simulink model "harness"  (Simulink 7.0)
settings: Solver=ode23  StartTime=0.0  StopTime=20  FixedStep=0.01  RelTol=1e-3
InitFcn:
  | init_simulation
StopFcn:
  | post_simulation
values from neighbouring files (symbols this model uses):
  A = pi*R^2    (= 0.0506707479097)    [constants.m]
  accel_noise = noise_on*.01^2    [constants.m]
  Alpha = pi/180*[-85:5:85]    [constants.m]
  att_noise = noise_on*(.25*pi/180)^2    [constants.m]
  att_ref = [0.2 0.2 0 0 0 0]'    [run_simulation.m]
  att_traj_on = 0    [set_scenario.m]
  b = 0.1    [constants.m]
  const_wind = [1 1 0]    [run_simulation.m]
  g = [0 0 9.8]'    [constants.m]
  gyro_noise = noise_on*.01^2    [constants.m]
  J = [Jxx 0 0 ... (first row only)    [constants.m]
  K_a1s = .009    (= 0.009)    [constants.m]
  K_attitude = [  0   kp_p   kp_y     0    kd_p   kd_y ... (first row only)    [run_simulation.m]
  K_beta = 0.23    [constants.m]
  K_dz = 0.7    [run_simulation.m]
  K_flap = 4*(K_beta + T_nom*dz)*K_a1s/(2*dx)    (= 0.0320793572835)    [constants.m]
  K_pz = .37    (= 0.37)    [run_simulation.m]
  K_torque = 0.47    [constants.m]
  M = 1.8263    [constants.m]
  motor_noise = noise_on*(9.8/4*.05)^2    [constants.m]
  plant_int_period = t_s / tau_motor    (= 0.00131578947368)    [constants.m]
  pos_noise = noise_on*0.02^2    [constants.m]
  r1 = [dx 0 -dz]'    [constants.m]
  r2 = [0 dx -dz]'    [constants.m]
  r3 = [-dx 0 -dz]'    [constants.m]
  r4 = [0 -dx -dz]'    [constants.m]
  R_90 = [0 -1 0 ... (first row only)    [constants.m]
  rho = 1.2    [constants.m]
  select = 0    [run_simulation.m]
  T_nom = M*9.8/4    (= 4.474435)    [constants.m]
  t_s = 1/76    (= 0.0131578947368)    [constants.m]
  tau_motor = 10    [constants.m]
  thrust_max = 9.8 * 1    (= 9.8)    [constants.m]
  thrust_min = 0    [constants.m]
  v_min = 1e-3    (= 0.001)    [constants.m]
  vel_noise = noise_on*0.05^2    [constants.m]
  Vh = sqrt(T/(2*rho*A))    [constants.m]
  Vinf = [0:0.5:6]    [constants.m]
  w_seed = 0    [run_simulation.m]
  wind = 3    [run_simulation.m]
  wind_clip = wind_max    (= 10)    [run_simulation.m]
  wind_duration = 5    [run_simulation.m]
  wind_max = 10    [run_simulation.m]
  wind_start = 3    [run_simulation.m]
  wind_var = (wind_max / 10)^2    (= 1)    [run_simulation.m]
  wind_vector = [1 0 0]'    [run_simulation.m]
  zd_ref = 0    [run_simulation.m]
undefined symbols (not defined in the file or in its folder): DiscIntNeverNeededParam, ToverTh
libraries: simulink x20
(part 1 of 3)
settings Model: Creator=Steve  LastModifiedBy=jporter  ExtModeAutoUpdateStatusClock=off
settings DebuggingCC: SaveWithParameterizedLinksMsg=none  SignalResolutionControl=TryResolveAllWithWarning  MultiTaskDSMMsg=warning  MultiTaskCondExecSysMsg=none  StrictBusMsg=None
settings RTWCC: IncludeERTFirstTime=on
settings GRTTargetCC: TargetFcnLib=ansi_tfl_tmw.mat

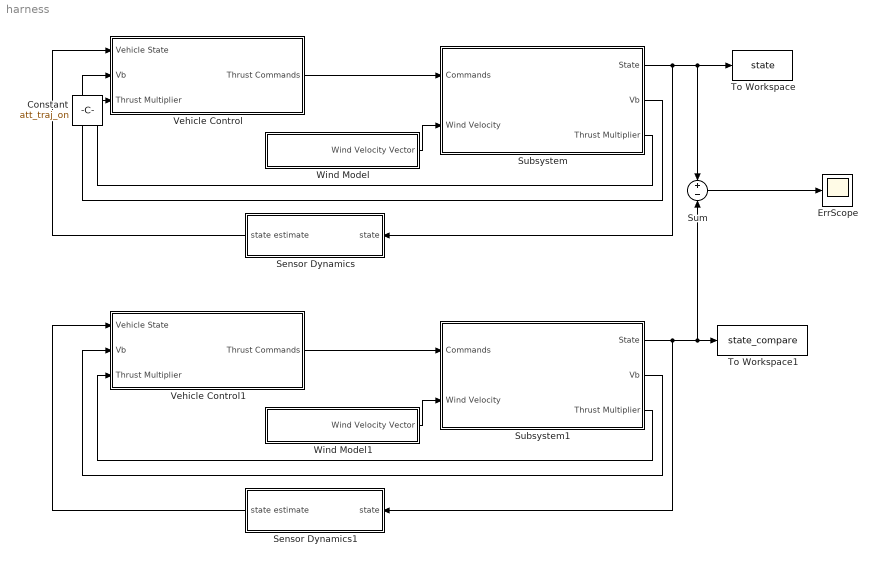
== system harness ==
  ErrScope : Scope
      settings: SaveName=ScopeData22
  Sensor Dynamics : Subsystem  Orientation=left
  Sensor Dynamics1 : Subsystem  Orientation=left
  Subsystem : Subsystem
  Subsystem1 : Subsystem
  Sum : Sum  Inputs=+|-  OutDataType=sfix(16)  OutScaling=2^0
  To Workspace : ToWorkspace  VariableName=state  SampleTime=-1  SaveFormat=Structure With Time
  To Workspace1 : ToWorkspace  VariableName=state_compare  SampleTime=-1  SaveFormat=Structure With Time
  Vehicle Control : Subsystem
  Vehicle Control1 : Subsystem
  Wind Model : Subsystem
  Wind Model1 : Subsystem
  Constant : Constant  IOType=siggen  Value=att_traj_on  OutDataType=sfix(16)  OutScaling=2^0
  wires:
  Wind Model/1(Wind Velocity Vector) -> Subsystem/2(Wind Velocity)
  Vehicle Control/1(Thrust Commands) -> Subsystem/1(Commands)
  Sensor Dynamics/1(state estimate) -> Vehicle Control/1(Vehicle State)
  Subsystem/1(State) -> Sensor Dynamics/1(state), To Workspace/1, Sum/1
  Subsystem/2(Vb) -> Vehicle Control/2(Vb)
  Subsystem/3(Thrust Multiplier) -> Vehicle Control/3(Thrust Multiplier)
  Wind Model1/1(Wind Velocity Vector) -> Subsystem1/2(Wind Velocity)
  Vehicle Control1/1(Thrust Commands) -> Subsystem1/1(Commands)
  Sensor Dynamics1/1(state estimate) -> Vehicle Control1/1(Vehicle State)
  Subsystem1/1(State) -> Sensor Dynamics1/1(state), To Workspace1/1, Sum/2
  Subsystem1/2(Vb) -> Vehicle Control1/2(Vb)
  Subsystem1/3(Thrust Multiplier) -> Vehicle Control1/3(Thrust Multiplier)
  Sum/1 -> ErrScope/1

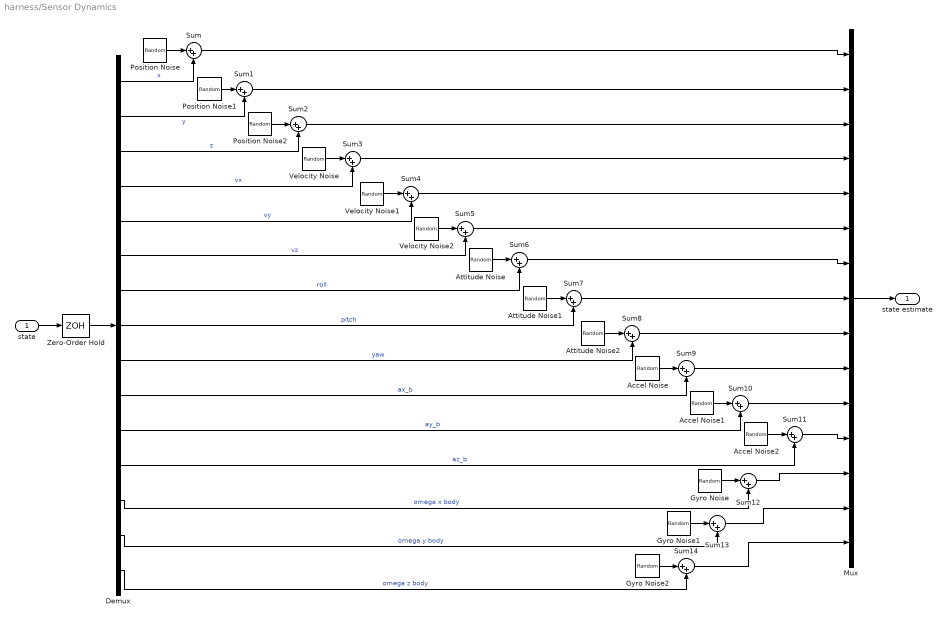
== system harness/Sensor Dynamics ==
  state : Inport  OutDataType=sfix(16)  OutScaling=2^0
  Accel Noise : RandomNumber  Variance=accel_noise  Seed=9  SampleTime=t_s
  Accel Noise1 : RandomNumber  Variance=accel_noise  Seed=10  SampleTime=t_s
  Accel Noise2 : RandomNumber  Variance=accel_noise  Seed=11  SampleTime=t_s
  Attitude Noise : RandomNumber  Variance=att_noise  Seed=6  SampleTime=t_s
  Attitude Noise1 : RandomNumber  Variance=att_noise  Seed=7  SampleTime=t_s
  Attitude Noise2 : RandomNumber  Variance=att_noise  Seed=8  SampleTime=t_s
  Demux : Demux  Outputs=15
  Gyro Noise : RandomNumber  Variance=gyro_noise  Seed=12  SampleTime=t_s
  Gyro Noise1 : RandomNumber  Variance=gyro_noise  Seed=13  SampleTime=t_s
  Gyro Noise2 : RandomNumber  Variance=gyro_noise  Seed=14  SampleTime=t_s
  Mux : Mux  Inputs=15
  Position Noise : RandomNumber  Variance=pos_noise  SampleTime=t_s
  Position Noise1 : RandomNumber  Variance=pos_noise  Seed=1  SampleTime=t_s
  Position Noise2 : RandomNumber  Variance=pos_noise  Seed=3  SampleTime=t_s
  Sum{,1..14} (15 alike) : Sum  Inputs=|++  OutDataType=sfix(16)  OutScaling=2^0
  Velocity Noise : RandomNumber  Variance=vel_noise  Seed=3  SampleTime=t_s
  Velocity Noise1 : RandomNumber  Variance=vel_noise  Seed=4  SampleTime=t_s
  Velocity Noise2 : RandomNumber  Variance=vel_noise  Seed=5  SampleTime=t_s
  Zero-Order Hold : ZeroOrderHold  SampleTime=t_s
  state estimate : Outport  OutDataType=sfix(16)  OutScaling=2^0
  wires:
  state/1 -> Zero-Order Hold/1
  Zero-Order Hold/1 -> Demux/1
  Demux/1 -> Sum/2  "x"
  Demux/2 -> Sum1/2  "y"
  Demux/5 -> Sum4/2  "vy"
  Demux/4 -> Sum3/2  "vx"
  Demux/7 -> Sum6/2  "roll"
  Demux/8 -> Sum7/2  "pitch"
  Demux/9 -> Sum8/2  "yaw"
  Demux/3 -> Sum2/2  "z"
  Demux/6 -> Sum5/2  "vz"
  Demux/10 -> Sum9/2  "ax_b"
  Demux/11 -> Sum10/2  "ay_b"
  Demux/12 -> Sum11/2  "az_b"
  Demux/14 -> Sum13/2  "omega y body"
  Demux/15 -> Sum14/2  "omega z body"
  Demux/13 -> Sum12/2  "omega x body"
  Position Noise/1 -> Sum/1
  Position Noise1/1 -> Sum1/1
  Position Noise2/1 -> Sum2/1
  Velocity Noise/1 -> Sum3/1
  Velocity Noise1/1 -> Sum4/1
  Velocity Noise2/1 -> Sum5/1
  Attitude Noise/1 -> Sum6/1
  Attitude Noise1/1 -> Sum7/1
  Attitude Noise2/1 -> Sum8/1
  Accel Noise/1 -> Sum9/1
  Accel Noise1/1 -> Sum10/1
  Accel Noise2/1 -> Sum11/1
  Gyro Noise/1 -> Sum12/1
  Gyro Noise1/1 -> Sum13/1
  Gyro Noise2/1 -> Sum14/1
  Sum/1 -> Mux/1
  Sum1/1 -> Mux/2
  Sum2/1 -> Mux/3
  Sum3/1 -> Mux/4
  Sum4/1 -> Mux/5
  Sum5/1 -> Mux/6
  Sum6/1 -> Mux/7
  Sum7/1 -> Mux/8
  Sum8/1 -> Mux/9
  Sum9/1 -> Mux/10
  Sum10/1 -> Mux/11
  Sum11/1 -> Mux/12
  Sum12/1 -> Mux/13
  Sum13/1 -> Mux/14
  Sum14/1 -> Mux/15
  Mux/1 -> state estimate/1

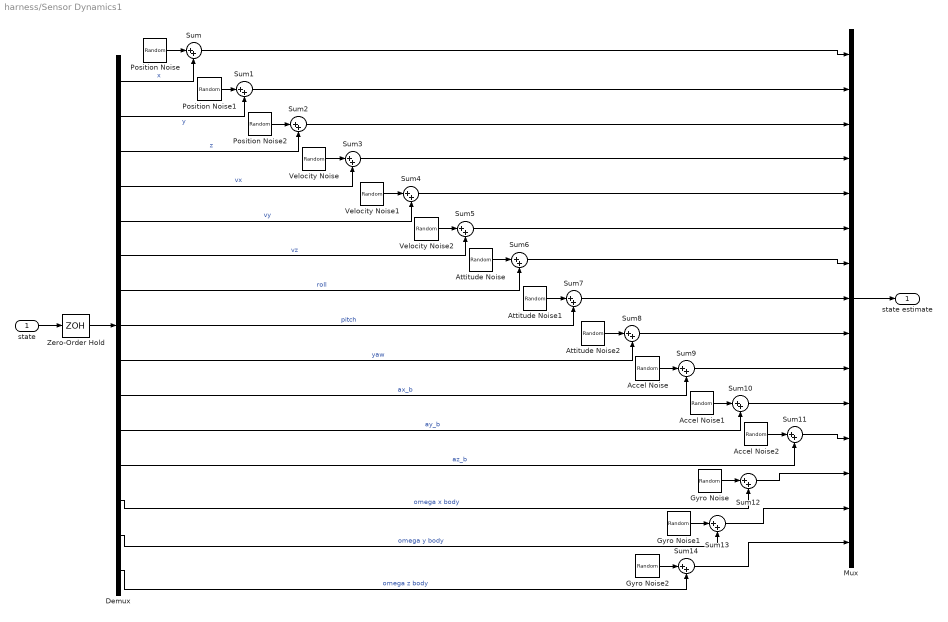
== system harness/Sensor Dynamics1 ==
  state : Inport  OutDataType=sfix(16)  OutScaling=2^0
  Accel Noise : RandomNumber  Variance=accel_noise  Seed=9  SampleTime=t_s
  Accel Noise1 : RandomNumber  Variance=accel_noise  Seed=10  SampleTime=t_s
  Accel Noise2 : RandomNumber  Variance=accel_noise  Seed=11  SampleTime=t_s
  Attitude Noise : RandomNumber  Variance=att_noise  Seed=6  SampleTime=t_s
  Attitude Noise1 : RandomNumber  Variance=att_noise  Seed=7  SampleTime=t_s
  Attitude Noise2 : RandomNumber  Variance=att_noise  Seed=8  SampleTime=t_s
  Demux : Demux  Outputs=15
  Gyro Noise : RandomNumber  Variance=gyro_noise  Seed=12  SampleTime=t_s
  Gyro Noise1 : RandomNumber  Variance=gyro_noise  Seed=13  SampleTime=t_s
  Gyro Noise2 : RandomNumber  Variance=gyro_noise  Seed=14  SampleTime=t_s
  Mux : Mux  Inputs=15
  Position Noise : RandomNumber  Variance=pos_noise  SampleTime=t_s
  Position Noise1 : RandomNumber  Variance=pos_noise  Seed=1  SampleTime=t_s
  Position Noise2 : RandomNumber  Variance=pos_noise  Seed=3  SampleTime=t_s
  Sum{,1..14} (15 alike) : Sum  Inputs=|++  OutDataType=sfix(16)  OutScaling=2^0
  Velocity Noise : RandomNumber  Variance=vel_noise  Seed=3  SampleTime=t_s
  Velocity Noise1 : RandomNumber  Variance=vel_noise  Seed=4  SampleTime=t_s
  Velocity Noise2 : RandomNumber  Variance=vel_noise  Seed=5  SampleTime=t_s
  Zero-Order Hold : ZeroOrderHold  SampleTime=t_s
  state estimate : Outport  OutDataType=sfix(16)  OutScaling=2^0
  wires:
  state/1 -> Zero-Order Hold/1
  Zero-Order Hold/1 -> Demux/1
  Demux/1 -> Sum/2  "x"
  Demux/2 -> Sum1/2  "y"
  Demux/5 -> Sum4/2  "vy"
  Demux/4 -> Sum3/2  "vx"
  Demux/7 -> Sum6/2  "roll"
  Demux/8 -> Sum7/2  "pitch"
  Demux/9 -> Sum8/2  "yaw"
  Demux/3 -> Sum2/2  "z"
  Demux/6 -> Sum5/2  "vz"
  Demux/10 -> Sum9/2  "ax_b"
  Demux/11 -> Sum10/2  "ay_b"
  Demux/12 -> Sum11/2  "az_b"
  Demux/14 -> Sum13/2  "omega y body"
  Demux/15 -> Sum14/2  "omega z body"
  Demux/13 -> Sum12/2  "omega x body"
  Position Noise/1 -> Sum/1
  Position Noise1/1 -> Sum1/1
  Position Noise2/1 -> Sum2/1
  Velocity Noise/1 -> Sum3/1
  Velocity Noise1/1 -> Sum4/1
  Velocity Noise2/1 -> Sum5/1
  Attitude Noise/1 -> Sum6/1
  Attitude Noise1/1 -> Sum7/1
  Attitude Noise2/1 -> Sum8/1
  Accel Noise/1 -> Sum9/1
  Accel Noise1/1 -> Sum10/1
  Accel Noise2/1 -> Sum11/1
  Gyro Noise/1 -> Sum12/1
  Gyro Noise1/1 -> Sum13/1
  Gyro Noise2/1 -> Sum14/1
  Sum/1 -> Mux/1
  Sum1/1 -> Mux/2
  Sum2/1 -> Mux/3
  Sum3/1 -> Mux/4
  Sum4/1 -> Mux/5
  Sum5/1 -> Mux/6
  Sum6/1 -> Mux/7
  Sum7/1 -> Mux/8
  Sum8/1 -> Mux/9
  Sum9/1 -> Mux/10
  Sum10/1 -> Mux/11
  Sum11/1 -> Mux/12
  Sum12/1 -> Mux/13
  Sum13/1 -> Mux/14
  Sum14/1 -> Mux/15
  Mux/1 -> state estimate/1

== system harness/Subsystem ==
  Commands : Inport  OutDataType=sfix(16)  OutScaling=2^0
  Wind Velocity : Inport  Port=2  OutDataType=sfix(16)  OutScaling=2^0
  6DOF (Euler Angles)_CMU : Subsystem
  Aerodynamic Effects : Subsystem
  Gravity : Constant  Value=g * M  OutDataType=sfix(16)  OutScaling=2^0
  Moments : Scope
      settings: SaveName=ScopeData7
  Motor Dynamics : Subsystem
  Mux : Mux  Inputs=5
  Product : Product  Multiplication=Matrix(*)  OutDataType=sfix(16)  OutScaling=2^0  RndMeth=Zero
  Product1 : Product  Multiplication=Matrix(*)  OutDataType=sfix(16)  OutScaling=2^0  RndMeth=Zero
  Sum : Sum  Inputs=|+++  OutDataType=sfix(16)  OutScaling=2^0
  Sum1 : Sum  Inputs=|+-  OutDataType=sfix(16)  OutScaling=2^0
  Terminator : Terminator
  Thrusts actual : Scope
      settings: SaveName=ScopeData9
  Viscous Drag : Gain  Gain=-b  ParameterDataType=sfix(16)  ParameterScaling=2^0  OutDataType=sfix(16)  OutScaling=2^0
  Zero-Order Hold : ZeroOrderHold  SampleTime=t_s
  State : Outport  OutDataType=sfix(16)  OutScaling=2^0
  Vb : Outport  Port=2  OutDataType=sfix(16)  OutScaling=2^0
  Thrust Multiplier : Outport  Port=3  OutDataType=sfix(16)  OutScaling=2^0
  wires:
  Motor Dynamics/1(Motor Thrusts) -> Thrusts actual/1, Aerodynamic Effects/1(Thrusts)
  Product/1 -> Sum/1
  Sum/1 -> 6DOF (Euler Angles)_CMU/1(F_xyz(N))
  6DOF (Euler Angles)_CMU/4(DCM) -> Product/1, Product1/1
  Gravity/1 -> Product/2
  Sum1/1 -> Aerodynamic Effects/2("V (body, relative)"), Viscous Drag/1
  Product1/1 -> Sum1/2
  6DOF (Euler Angles)_CMU/5(Vb) -> Sum1/1, Vb/1
  Viscous Drag/1 -> Sum/3
  6DOF (Euler Angles)_CMU/2(Xe) -> Mux/1
  6DOF (Euler Angles)_CMU/1(Ve) -> Mux/2
  6DOF (Euler Angles)_CMU/3(Euler) -> Mux/3
  Aerodynamic Effects/2(Body Moments) -> Moments/1, 6DOF (Euler Angles)_CMU/2(M_xyz(Nm))
  Aerodynamic Effects/1(Thrust Forces) -> Sum/2
  Zero-Order Hold/1 -> Motor Dynamics/1(Motor Commands)
  Mux/1 -> State/1
  Commands/1 -> Zero-Order Hold/1
  Wind Velocity/1 -> Product1/2
  Aerodynamic Effects/3(Thrust Multiplier) -> Thrust Multiplier/1
  6DOF (Euler Angles)_CMU/7(pdot,qdot,rdot) -> Terminator/1
  6DOF (Euler Angles)_CMU/6(p,q,r) -> Mux/5
  6DOF (Euler Angles)_CMU/8(Ab) -> Mux/4

== system harness/Subsystem1 ==
  Commands : Inport  OutDataType=sfix(16)  OutScaling=2^0
  Wind Velocity : Inport  Port=2  OutDataType=sfix(16)  OutScaling=2^0
  6DOF (Euler Angles)_CMU : Subsystem
  Aerodynamic Effects : Subsystem
  Gravity : Constant  Value=g * M  OutDataType=sfix(16)  OutScaling=2^0
  Moments : Scope
      settings: SaveName=ScopeData7
  Motor Dynamics : Subsystem
  Mux : Mux  Inputs=5
  Product : Product  Multiplication=Matrix(*)  OutDataType=sfix(16)  OutScaling=2^0  RndMeth=Zero
  Product1 : Product  Multiplication=Matrix(*)  OutDataType=sfix(16)  OutScaling=2^0  RndMeth=Zero
  Sum : Sum  Inputs=|+++  OutDataType=sfix(16)  OutScaling=2^0
  Sum1 : Sum  Inputs=|+-  OutDataType=sfix(16)  OutScaling=2^0
  Terminator : Terminator
  Thrusts actual : Scope
      settings: SaveName=ScopeData9
  Viscous Drag : Gain  Gain=-b  ParameterDataType=sfix(16)  ParameterScaling=2^0  OutDataType=sfix(16)  OutScaling=2^0
  Zero-Order Hold : ZeroOrderHold  SampleTime=plant_int_period
  State : Outport  OutDataType=sfix(16)  OutScaling=2^0
  Vb : Outport  Port=2  OutDataType=sfix(16)  OutScaling=2^0
  Thrust Multiplier : Outport  Port=3  OutDataType=sfix(16)  OutScaling=2^0
  wires:
  Motor Dynamics/1(Motor Thrusts) -> Thrusts actual/1, Aerodynamic Effects/1(Thrusts)
  Product/1 -> Sum/1
  Sum/1 -> 6DOF (Euler Angles)_CMU/1(F_xyz(N))
  6DOF (Euler Angles)_CMU/4(DCM) -> Product/1, Product1/1
  Gravity/1 -> Product/2
  Sum1/1 -> Aerodynamic Effects/2("V (body, relative)"), Viscous Drag/1
  Product1/1 -> Sum1/2
  6DOF (Euler Angles)_CMU/5(Vb) -> Sum1/1, Vb/1
  Viscous Drag/1 -> Sum/3
  6DOF (Euler Angles)_CMU/2(Xe) -> Mux/1
  6DOF (Euler Angles)_CMU/1(Ve) -> Mux/2
  6DOF (Euler Angles)_CMU/3(Euler) -> Mux/3
  Aerodynamic Effects/2(Body Moments) -> Moments/1, 6DOF (Euler Angles)_CMU/2(M_xyz(Nm))
  Aerodynamic Effects/1(Thrust Forces) -> Sum/2
  Mux/1 -> State/1
  Commands/1 -> Motor Dynamics/1(Motor Commands)
  Wind Velocity/1 -> Zero-Order Hold/1
  Aerodynamic Effects/3(Thrust Multiplier) -> Thrust Multiplier/1
  6DOF (Euler Angles)_CMU/7(pdot,qdot,rdot) -> Terminator/1
  6DOF (Euler Angles)_CMU/6(p,q,r) -> Mux/5
  6DOF (Euler Angles)_CMU/8(Ab) -> Mux/4
  Zero-Order Hold/1 -> Product1/2

== system harness/Vehicle Control ==
  Vehicle State : Inport  OutDataType=sfix(16)  OutScaling=2^0
  Vb : Inport  Port=2  OutDataType=sfix(16)  OutScaling=2^0
  Thrust Multiplier : Inport  Port=3  OutDataType=sfix(16)  OutScaling=2^0
  Altitude Control : Subsystem
  Attitude Control : Subsystem
  Position Control : Subsystem
  Reference Altitude : FromWorkspace  VariableName=alt_traj  SampleTime=0
  Reference Attitude : FromWorkspace  VariableName=att_traj  SampleTime=0
  Scope : Scope
      settings: SaveName=ScopeData11
  Scope1 : Scope
      settings: SaveName=ScopeData12
  Sum : Sum  Inputs=|++  OutDataType=sfix(16)  OutScaling=2^0
  Switch : Switch
  Thrust Commands : Outport  OutDataType=sfix(16)  OutScaling=2^0
  wires:
  Vehicle State/1 -> Position Control/1(state), Attitude Control/2(State), Altitude Control/2(state)
  Attitude Control/1(Thrusts) -> Sum/1
  Position Control/1(Attitude) -> Switch/3
  Switch/1 -> Attitude Control/1(Attitude Commands)
  Reference Attitude/1 -> Scope/1, Switch/1
  Sum/1 -> Thrust Commands/1
  Altitude Control/1(commands) -> Sum/2
  Reference Altitude/1 -> Scope1/1, Altitude Control/1(altitude  commands)
  Vb/1 -> Attitude Control/3(Vb)
  Thrust Multiplier/1 -> Altitude Control/3(Thrust Multiplier)

== system harness/Vehicle Control1 ==
  Vehicle State : Inport  OutDataType=sfix(16)  OutScaling=2^0
  Vb : Inport  Port=2  OutDataType=sfix(16)  OutScaling=2^0
  Thrust Multiplier : Inport  Port=3  OutDataType=sfix(16)  OutScaling=2^0
  Altitude Control : Subsystem
  Attitude Control : Subsystem
  Constant : Constant  Value=att_traj_on  OutDataType=sfix(16)  OutScaling=2^0
  Position Control : Subsystem
  Reference Altitude : FromWorkspace  VariableName=alt_traj  SampleTime=0
  Reference Attitude : FromWorkspace  VariableName=att_traj  SampleTime=0
  Scope : Scope
      settings: SaveName=ScopeData11
  Scope1 : Scope
      settings: SaveName=ScopeData12
  Sum : Sum  Inputs=|++  OutDataType=sfix(16)  OutScaling=2^0
  Switch : Switch
  Zero-Order Hold : ZeroOrderHold  SampleTime=t_s
  Thrust Commands : Outport  OutDataType=sfix(16)  OutScaling=2^0
  wires:
  Vehicle State/1 -> Position Control/1(state), Attitude Control/2(State), Altitude Control/2(state)
  Attitude Control/1(Thrusts) -> Sum/1
  Position Control/1(Attitude) -> Switch/3
  Switch/1 -> Attitude Control/1(Attitude Commands)
  Reference Attitude/1 -> Switch/1, Scope/1
  Sum/1 -> Zero-Order Hold/1
  Altitude Control/1(commands) -> Sum/2
  Reference Altitude/1 -> Scope1/1, Altitude Control/1(altitude  commands)
  Vb/1 -> Attitude Control/3(Vb)
  Thrust Multiplier/1 -> Altitude Control/3(Thrust Multiplier)
  Zero-Order Hold/1 -> Thrust Commands/1
  Constant/1 -> Switch/2

== system harness/Wind Model ==
  Constant : Constant  Value=wind  OutDataType=sfix(16)  OutScaling=2^0
  Constant wind : Constant  Value=const_wind  OutDataType=sfix(16)  OutScaling=2^0
  Multiport Switch : MultiPortSwitch  Inputs=3
  Single Wind Gust Model : Subsystem  TreatAsAtomicUnit=on
  Step : Step  Time=wind_start  SampleTime=0
  Step1 : Step  Time=wind_start+wind_duration  After=-1  SampleTime=0
  Sum : Sum  Inputs=|++  OutDataType=sfix(16)  OutScaling=2^0
  Zero Wind : Constant  Value=[0 0 0]'  OutDataType=sfix(16)  OutScaling=2^0
  wind : Scope
      settings: SaveName=ScopeData4
  Wind Velocity Vector : Outport  OutDataType=sfix(16)  OutScaling=2^0
  wires:
  Multiport Switch/1 -> Wind Velocity Vector/1, wind/1
  Step/1 -> Sum/1  "start"
  Step1/1 -> Sum/2  "stop"
  Sum/1 -> Single Wind Gust Model/Enable
  Constant/1 -> Multiport Switch/1
  Zero Wind/1 -> Multiport Switch/2
  Constant wind/1 -> Multiport Switch/3
  Single Wind Gust Model/1(Wind Velocity) -> Multiport Switch/4

== system harness/Wind Model1 ==
  Constant : Constant  Value=wind  OutDataType=sfix(16)  OutScaling=2^0
  Constant wind : Constant  Value=const_wind  OutDataType=sfix(16)  OutScaling=2^0
  Multiport Switch : MultiPortSwitch  Inputs=3
  Single Wind Gust Model : Subsystem  TreatAsAtomicUnit=on
  Step : Step  Time=wind_start  SampleTime=0
  Step1 : Step  Time=wind_start+wind_duration  After=-1  SampleTime=0
  Sum : Sum  Inputs=|++  OutDataType=sfix(16)  OutScaling=2^0
  Zero Wind : Constant  Value=[0 0 0]'  OutDataType=sfix(16)  OutScaling=2^0
  wind : Scope
      settings: SaveName=ScopeData4
  Wind Velocity Vector : Outport  OutDataType=sfix(16)  OutScaling=2^0
  wires:
  Multiport Switch/1 -> Wind Velocity Vector/1, wind/1
  Step/1 -> Sum/1  "start"
  Step1/1 -> Sum/2  "stop"
  Sum/1 -> Single Wind Gust Model/Enable
  Constant/1 -> Multiport Switch/1
  Zero Wind/1 -> Multiport Switch/2
  Constant wind/1 -> Multiport Switch/3
  Single Wind Gust Model/1(Wind Velocity) -> Multiport Switch/4

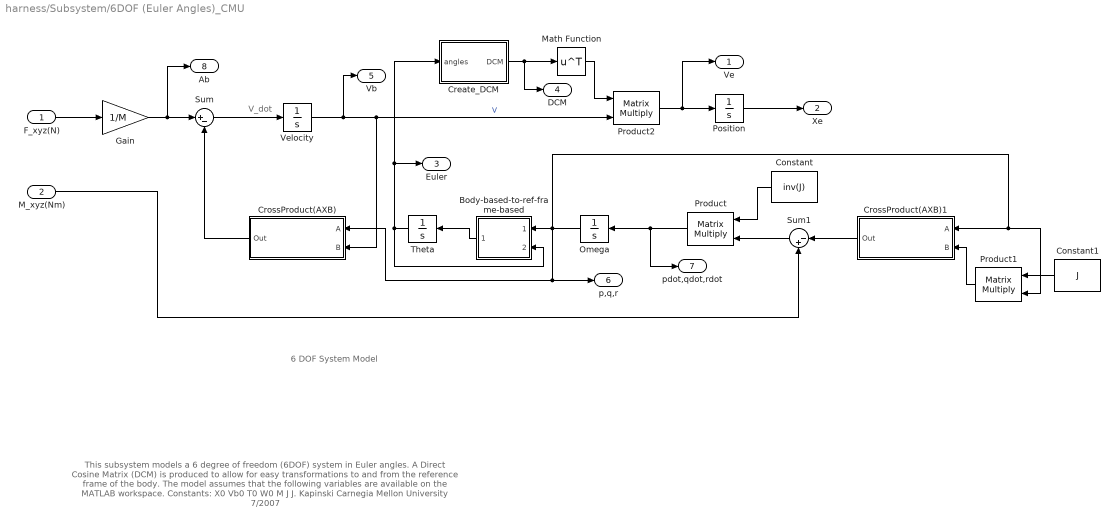
== system harness/Subsystem/6DOF (Euler Angles)_CMU ==
  note: 6 DOF System Model
  note: V_dot
  note: This subsystem models a 6 degree of freedom (6DOF) system in Euler angles.
      | A Direct Cosine Matrix (DCM) is produced to allow for easy transformations to
      | and from the reference frame of the body.  The model assumes that the
      | following variables are available on the MATLAB workspace.
      |
      | Constants:
      | X0
      | Vb0
      | T0
      | W0
      | M
      | J
      |
      | J. Kapinski
      | Carnegia Mellon University
      | 7/2007
  F_xyz(N) : Inport  OutDataType=sfix(16)  OutScaling=2^0
  M_xyz(Nm) : Inport  Port=2  PortDimensions=3  OutDataType=sfix(16)  OutScaling=2^0
  Body-based-to-ref-frame-based : Subsystem  Orientation=left
  Constant : Constant  Orientation=left  Value=inv(J)  OutDataType=sfix(16)  OutScaling=2^0
  Constant1 : Constant  Orientation=left  Value=J  OutDataType=sfix(16)  OutScaling=2^0
  Create_DCM : Subsystem
  CrossProduct(AXB) : Subsystem  Orientation=left
  CrossProduct(AXB)1 : Subsystem  Orientation=left
  Gain : Gain  Gain=1/M  ParameterDataType=sfix(16)  ParameterScaling=2^0  OutDataType=sfix(16)  OutScaling=2^0
  Math Function : Math  Operator=transpose  OutDataType=sfix(16)  OutScaling=2^0  SaturateOnIntegerOverflow=on
  Omega : Integrator  Orientation=left
  Position : Integrator
  Product : Product  Orientation=left  Multiplication=Matrix(*)  OutDataType=sfix(16)  OutScaling=2^0  RndMeth=Zero
  Product1 : Product  Orientation=left  Multiplication=Matrix(*)  OutDataType=sfix(16)  OutScaling=2^0  RndMeth=Zero
  Product2 : Product  Multiplication=Matrix(*)  OutDataType=sfix(16)  OutScaling=2^0  RndMeth=Zero
  Sum : Sum  Inputs=|+-  OutDataType=sfix(16)  OutScaling=2^0
  Sum1 : Sum  Orientation=left  Inputs=|-+  OutDataType=sfix(16)  OutScaling=2^0
  Theta : Integrator  Orientation=left
  Velocity : Integrator
  Ve : Outport  OutDataType=sfix(16)  OutScaling=2^0
  Xe : Outport  Port=2  OutDataType=sfix(16)  OutScaling=2^0
  Euler : Outport  Port=3  OutDataType=sfix(16)  OutScaling=2^0
  DCM : Outport  Port=4  OutDataType=sfix(16)  OutScaling=2^0
  Vb : Outport  Port=5  OutDataType=sfix(16)  OutScaling=2^0
  p,q,r : Outport  Port=6  OutDataType=sfix(16)  OutScaling=2^0
  pdot,qdot,rdot : Outport  Port=7  OutDataType=sfix(16)  OutScaling=2^0
  Ab : Outport  Port=8  OutDataType=sfix(16)  OutScaling=2^0
  wires:
  Position/1 -> Xe/1
  Product2/1 -> Ve/1, Position/1
  Math Function/1 -> Product2/1
  Create_DCM/1(DCM) -> DCM/1, Math Function/1
  Body-based-to-ref-frame-based/1(Out1) -> Theta/1
  Theta/1 -> Euler/1, Create_DCM/1(angles), Body-based-to-ref-frame-based/2(theta)
  Product1/1 -> CrossProduct(AXB)1/2(B)
  Constant1/1 -> Product1/1
  CrossProduct(AXB)1/1(Out) -> Sum1/1
  M_xyz(Nm)/1 -> Sum1/2
  Sum1/1 -> Product/2
  Product/1 -> pdot,qdot,rdot/1, Omega/1
  Constant/1 -> Product/1
  Velocity/1 -> Vb/1, Product2/2, CrossProduct(AXB)/2(B)  "V"
  Omega/1 -> p,q,r/1, CrossProduct(AXB)/1(A), Body-based-to-ref-frame-based/1(omega), Product1/2, CrossProduct(AXB)1/1(A)
  Sum/1 -> Velocity/1
  CrossProduct(AXB)/1(Out) -> Sum/2
  Gain/1 -> Ab/1, Sum/1
  F_xyz(N)/1 -> Gain/1

== system harness/Subsystem/Aerodynamic Effects ==
  Thrusts : Inport  OutDataType=sfix(16)  OutScaling=2^0
  "V (body, relative)" : Inport  Port=2  OutDataType=sfix(16)  OutScaling=2^0
  Flapping Dynamics : Subsystem
  Moments : Subsystem
  Pick First 2 Elements : Constant  Value=[1 0 0; 0 1 0; 0 0 0]  OutDataType=sfix(16)  OutScaling=2^0
  Product : Product  OutDataType=sfix(16)  OutScaling=2^0  RndMeth=Zero
  Product2 : Product  Multiplication=Matrix(*)  OutDataType=sfix(16)  OutScaling=2^0  RndMeth=Zero
  Product4 : Product  OutDataType=sfix(16)  OutScaling=2^0  RndMeth=Zero
  Sum : Sum  Inputs=|++  OutDataType=sfix(16)  OutScaling=2^0
  Sum of Elements : Sum  Inputs=+  OutDataType=sfix(16)  OutScaling=2^-10
  Vertical Effect Dynamics : Subsystem
  Thrust Forces : Outport  OutDataType=sfix(16)  OutScaling=2^0
  Body Moments : Outport  Port=2  OutDataType=sfix(16)  OutScaling=2^0
  Thrust Multiplier : Outport  Port=3  OutDataType=sfix(16)  OutScaling=2^0
  wires:
  Thrusts/1 -> Product/1, Vertical Effect Dynamics/1(Thrust Command)
  Vertical Effect Dynamics/1(Thrust Multiplier) -> Product/2, Thrust Multiplier/1
  Product/1 -> Sum of Elements/1, Moments/1(Thrust Magnitudes)
  Pick First 2 Elements/1 -> Product2/1
  "V (body, relative)"/1 -> Product2/2, Vertical Effect Dynamics/2(V (body))
  Product2/1 -> Flapping Dynamics/1(Vb2_hat)
  Sum of Elements/1 -> Product4/1
  Product4/1 -> Thrust Forces/1
  Flapping Dynamics/1(thrust vector) -> Moments/2(Thrust Vector), Product4/2
  Moments/1(Body Moments) -> Sum/1
  Sum/1 -> Body Moments/1
  Flapping Dynamics/2(rotor blade moments) -> Sum/2

== system harness/Subsystem/Motor Dynamics ==
  Motor Commands : Inport  OutDataType=sfix(16)  OutScaling=2^0
  Demux : Demux
  Motor Noise Source : Subsystem
  Mux : Mux
  Saturation{,1..3} (4 alike) : Saturate  UpperLimit=thrust_max  LowerLimit=thrust_min
  Scope : Scope
      settings: SaveName=ScopeData8
  State-Space : StateSpace  A=-tau_motor*eye(4)  B=tau_motor*eye(4)  C=eye(4)  D=zeros(4,4)  X0=T_nom*ones(4,1)
  Sum{,1..3} (4 alike) : Sum  Inputs=|++  OutDataType=sfix(16)  OutScaling=2^0
  Motor Thrusts : Outport  OutDataType=sfix(16)  OutScaling=2^0
  wires:
  Demux/1 -> Saturation/1
  Demux/3 -> Saturation2/1
  Mux/1 -> Motor Thrusts/1
  Saturation/1 -> Sum/1
  Sum/1 -> Mux/1
  Saturation1/1 -> Sum2/1
  Sum2/1 -> Mux/2
  Saturation2/1 -> Sum3/1
  Sum3/1 -> Mux/3
  Saturation3/1 -> Sum1/1
  Sum1/1 -> Mux/4
  Motor Noise Source/1(Motor 1) -> Sum/2
  Motor Noise Source/2(Motor 2) -> Sum2/2
  Motor Noise Source/3(Motor 3) -> Sum3/2
  Motor Noise Source/4(Motor 4) -> Sum1/2
  Motor Commands/1 -> State-Space/1, Scope/1
  State-Space/1 -> Demux/1
  Demux/2 -> Saturation1/1
  Demux/4 -> Saturation3/1

== system harness/Subsystem1/6DOF (Euler Angles)_CMU ==
  note: 6 DOF System Model
  note: V_dot
  note: This subsystem models a 6 degree of freedom (6DOF) system in Euler angles.
      | A Direct Cosine Matrix (DCM) is produced to allow for easy transformations to
      | and from the reference frame of the body.  The model assumes that the
      | following variables are available on the MATLAB workspace.
      |
      | Constants:
      | X0
      | Vb0
      | T0
      | W0
      | M
      | J
      |
      | J. Kapinski
      | Carnegia Mellon University
      | 7/2007
  F_xyz(N) : Inport  OutDataType=sfix(16)  OutScaling=2^0
  M_xyz(Nm) : Inport  Port=2  PortDimensions=3  OutDataType=sfix(16)  OutScaling=2^0
  Body-based-to-ref-frame-based : Subsystem  Orientation=left
  Constant : Constant  Orientation=left  Value=inv(J)  OutDataType=sfix(16)  OutScaling=2^0
  Constant1 : Constant  Orientation=left  Value=J  OutDataType=sfix(16)  OutScaling=2^0
  Create_DCM : Subsystem
  CrossProduct(AXB) : Subsystem  Orientation=left
  CrossProduct(AXB)1 : Subsystem  Orientation=left
  Discrete-Time Omega : DiscreteIntegrator  Orientation=left  SampleTime=plant_int_period  OutDataType=sfix(16)  OutScaling=2^0  ICPrevOutput=DiscIntNeverNeededParam  ICPrevScaledInput=DiscIntNeverNeededParam
  Discrete-Time Position : DiscreteIntegrator  SampleTime=plant_int_period  OutDataType=sfix(16)  OutScaling=2^0  ICPrevOutput=DiscIntNeverNeededParam  ICPrevScaledInput=DiscIntNeverNeededParam
  Discrete-Time Theta : DiscreteIntegrator  Orientation=left  SampleTime=plant_int_period  OutDataType=sfix(16)  OutScaling=2^0  ICPrevOutput=DiscIntNeverNeededParam  ICPrevScaledInput=DiscIntNeverNeededParam
  Discrete-Time Velocity : DiscreteIntegrator  SampleTime=plant_int_period  OutDataType=sfix(16)  OutScaling=2^0  ICPrevOutput=DiscIntNeverNeededParam  ICPrevScaledInput=DiscIntNeverNeededParam
  Gain : Gain  Gain=1/M  ParameterDataType=sfix(16)  ParameterScaling=2^0  OutDataType=sfix(16)  OutScaling=2^0
  Math Function : Math  Operator=transpose  OutDataType=sfix(16)  OutScaling=2^0  SaturateOnIntegerOverflow=on
  Product : Product  Orientation=left  Multiplication=Matrix(*)  OutDataType=sfix(16)  OutScaling=2^0  RndMeth=Zero
  Product1 : Product  Orientation=left  Multiplication=Matrix(*)  OutDataType=sfix(16)  OutScaling=2^0  RndMeth=Zero
  Product2 : Product  Multiplication=Matrix(*)  OutDataType=sfix(16)  OutScaling=2^0  RndMeth=Zero
  Sum : Sum  Inputs=|+-  OutDataType=sfix(16)  OutScaling=2^0
  Sum1 : Sum  Orientation=left  Inputs=|-+  OutDataType=sfix(16)  OutScaling=2^0
  Ve : Outport  OutDataType=sfix(16)  OutScaling=2^0
  Xe : Outport  Port=2  OutDataType=sfix(16)  OutScaling=2^0
  Euler : Outport  Port=3  OutDataType=sfix(16)  OutScaling=2^0
  DCM : Outport  Port=4  OutDataType=sfix(16)  OutScaling=2^0
  Vb : Outport  Port=5  OutDataType=sfix(16)  OutScaling=2^0
  p,q,r : Outport  Port=6  OutDataType=sfix(16)  OutScaling=2^0
  pdot,qdot,rdot : Outport  Port=7  OutDataType=sfix(16)  OutScaling=2^0
  Ab : Outport  Port=8  OutDataType=sfix(16)  OutScaling=2^0
  wires:
  Discrete-Time Position/1 -> Xe/1
  Product2/1 -> Ve/1, Discrete-Time Position/1
  Math Function/1 -> Product2/1
  Create_DCM/1(DCM) -> DCM/1, Math Function/1
  Body-based-to-ref-frame-based/1(Out1) -> Discrete-Time Theta/1
  Discrete-Time Theta/1 -> Euler/1, Create_DCM/1(angles), Body-based-to-ref-frame-based/2(theta)
  Product1/1 -> CrossProduct(AXB)1/2(B)
  Constant1/1 -> Product1/1
  CrossProduct(AXB)1/1(Out) -> Sum1/1
  M_xyz(Nm)/1 -> Sum1/2
  Sum1/1 -> Product/2
  Product/1 -> pdot,qdot,rdot/1, Discrete-Time Omega/1
  Constant/1 -> Product/1
  Discrete-Time Velocity/1 -> Vb/1, Product2/2, CrossProduct(AXB)/2(B)  "V"
  Discrete-Time Omega/1 -> p,q,r/1, CrossProduct(AXB)/1(A), Body-based-to-ref-frame-based/1(omega), Product1/2, CrossProduct(AXB)1/1(A)
  Sum/1 -> Discrete-Time Velocity/1
  CrossProduct(AXB)/1(Out) -> Sum/2
  Gain/1 -> Ab/1, Sum/1
  F_xyz(N)/1 -> Gain/1

== system harness/Subsystem1/Aerodynamic Effects ==
  Thrusts : Inport  OutDataType=sfix(16)  OutScaling=2^0
  "V (body, relative)" : Inport  Port=2  OutDataType=sfix(16)  OutScaling=2^0
  Flapping Dynamics : Subsystem
  Moments : Subsystem
  Pick First 2 Elements : Constant  Value=[1 0 0; 0 1 0; 0 0 0]  OutDataType=sfix(16)  OutScaling=2^0
  Product : Product  OutDataType=sfix(16)  OutScaling=2^0  RndMeth=Zero
  Product2 : Product  Multiplication=Matrix(*)  OutDataType=sfix(16)  OutScaling=2^0  RndMeth=Zero
  Product4 : Product  OutDataType=sfix(16)  OutScaling=2^0  RndMeth=Zero
  Sum : Sum  Inputs=|++  OutDataType=sfix(16)  OutScaling=2^0
  Sum of Elements : Sum  Inputs=+  OutDataType=sfix(16)  OutScaling=2^-10
  Vertical Effect Dynamics : Subsystem
  Thrust Forces : Outport  OutDataType=sfix(16)  OutScaling=2^0
  Body Moments : Outport  Port=2  OutDataType=sfix(16)  OutScaling=2^0
  Thrust Multiplier : Outport  Port=3  OutDataType=sfix(16)  OutScaling=2^0
  wires:
  Thrusts/1 -> Product/1, Vertical Effect Dynamics/1(Thrust Command)
  Vertical Effect Dynamics/1(Thrust Multiplier) -> Product/2, Thrust Multiplier/1
  Product/1 -> Sum of Elements/1, Moments/1(Thrust Magnitudes)
  Pick First 2 Elements/1 -> Product2/1
  "V (body, relative)"/1 -> Product2/2, Vertical Effect Dynamics/2(V (body))
  Product2/1 -> Flapping Dynamics/1(Vb2_hat)
  Sum of Elements/1 -> Product4/1
  Product4/1 -> Thrust Forces/1
  Flapping Dynamics/1(thrust vector) -> Moments/2(Thrust Vector), Product4/2
  Moments/1(Body Moments) -> Sum/1
  Sum/1 -> Body Moments/1
  Flapping Dynamics/2(rotor blade moments) -> Sum/2

== system harness/Subsystem1/Motor Dynamics ==
  Motor Commands : Inport  OutDataType=sfix(16)  OutScaling=2^0
  Demux : Demux
  Discrete State-Space : DiscreteStateSpace  A=expm( -(tau_motor*plant_int_period) * eye(4) )  B=inv(expm( tau_motor * plant_int_period* eye(4))) * (expm((tau_motor*plant_int_period) * eye(4)) - eye(4))  C=eye(4)  D=zeros(4)  X0=T_nom * ones(4,1)  SampleTime=plant_int_period
  Motor Noise Source : Subsystem
  Mux : Mux
  Saturation{,1..3} (4 alike) : Saturate  UpperLimit=thrust_max  LowerLimit=thrust_min
  Scope : Scope
      settings: SaveName=ScopeData8
  Sum{,1..3} (4 alike) : Sum  Inputs=|++  OutDataType=sfix(16)  OutScaling=2^0
  Motor Thrusts : Outport  OutDataType=sfix(16)  OutScaling=2^0
  wires:
  Demux/1 -> Saturation/1
  Demux/3 -> Saturation2/1
  Mux/1 -> Motor Thrusts/1
  Saturation/1 -> Sum/1
  Sum/1 -> Mux/1
  Saturation1/1 -> Sum2/1
  Sum2/1 -> Mux/2
  Saturation2/1 -> Sum3/1
  Sum3/1 -> Mux/3
  Saturation3/1 -> Sum1/1
  Sum1/1 -> Mux/4
  Motor Noise Source/1(Motor 1) -> Sum/2
  Motor Noise Source/2(Motor 2) -> Sum2/2
  Motor Noise Source/3(Motor 3) -> Sum3/2
  Motor Noise Source/4(Motor 4) -> Sum1/2
  Motor Commands/1 -> Scope/1, Discrete State-Space/1
  Discrete State-Space/1 -> Demux/1
  Demux/2 -> Saturation1/1
  Demux/4 -> Saturation3/1

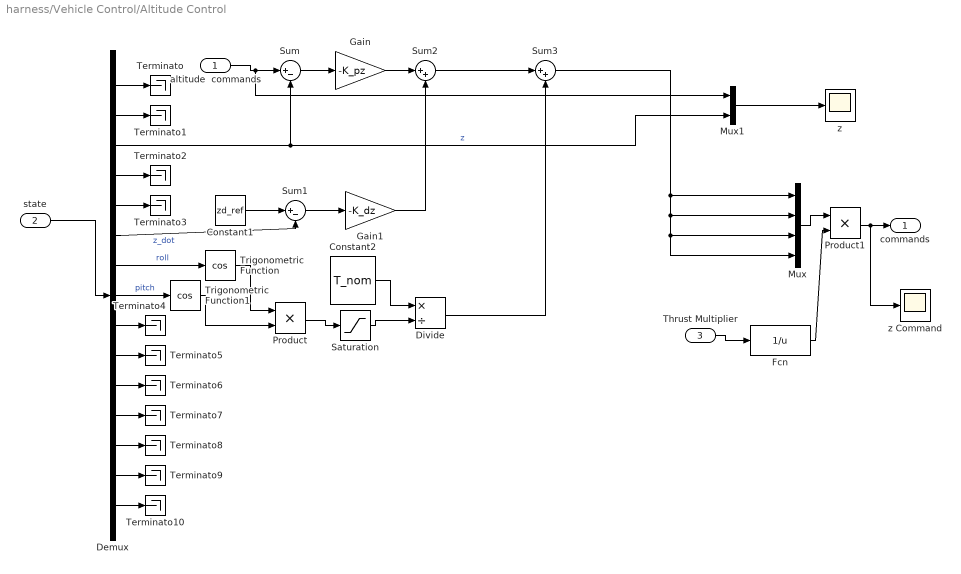
== system harness/Vehicle Control/Altitude Control ==
  altitude  commands : Inport  OutDataType=sfix(16)  OutScaling=2^0
  state : Inport  Port=2  OutDataType=sfix(16)  OutScaling=2^0
  Thrust Multiplier : Inport  Port=3  OutDataType=sfix(16)  OutScaling=2^0
  Constant1 : Constant  Value=zd_ref  OutDataType=sfix(16)  OutScaling=2^0
  Constant2 : Constant  Value=T_nom  OutDataType=sfix(16)  OutScaling=2^0
  Demux : Demux  Outputs=15
  Divide : Product  Inputs=*/  OutDataType=sfix(16)  OutScaling=2^-10
  Fcn : Fcn  Expr=1/u
  Gain : Gain  Gain=-K_pz  ParameterDataType=sfix(16)  ParameterScaling=2^0  OutDataType=sfix(16)  OutScaling=2^0
  Gain1 : Gain  Gain=-K_dz  ParameterDataType=sfix(16)  ParameterScaling=2^0  OutDataType=sfix(16)  OutScaling=2^0
  Mux : Mux
  Mux1 : Mux  Inputs=2
  Product : Product  OutDataType=sfix(16)  OutScaling=2^0  RndMeth=Zero
  Product1 : Product  OutDataType=sfix(16)  OutScaling=2^0  RndMeth=Zero
  Saturation : Saturate  UpperLimit=1  LowerLimit=0.01
  Sum : Sum  Inputs=|+-  OutDataType=sfix(16)  OutScaling=2^0
  Sum1 : Sum  Inputs=|+-  OutDataType=sfix(16)  OutScaling=2^0
  Sum2 : Sum  Inputs=|++  OutDataType=sfix(16)  OutScaling=2^0
  Sum3 : Sum  Inputs=|++  OutDataType=sfix(16)  OutScaling=2^0
  Terminato{,1..10} (11 alike) : Terminator
  Trigonometric Function : Trigonometry  Operator=cos
  Trigonometric Function1 : Trigonometry  Operator=cos
  z : Scope
      settings: SaveName=ScopeData3
  z Command : Scope
      settings: SaveName=ScopeData5
  commands : Outport  OutDataType=sfix(16)  OutScaling=2^0
  wires:
  state/1 -> Demux/1
  Demux/1 -> Terminato/1
  Demux/2 -> Terminato1/1
  Demux/5 -> Terminato3/1
  Demux/4 -> Terminato2/1
  Demux/3 -> Sum/2, Mux1/2  "z"
  altitude  commands/1 -> Sum/1, Mux1/1
  Constant1/1 -> Sum1/1
  Demux/6 -> Sum1/2  "z_dot"
  Sum/1 -> Gain/1
  Sum1/1 -> Gain1/1
  Gain/1 -> Sum2/1
  Gain1/1 -> Sum2/2
  Demux/7 -> Trigonometric Function/1  "roll"
  Demux/8 -> Trigonometric Function1/1  "pitch"
  Demux/9 -> Terminato4/1
  Trigonometric Function/1 -> Product/1
  Trigonometric Function1/1 -> Product/2
  Product/1 -> Saturation/1
  Constant2/1 -> Divide/1
  Sum2/1 -> Sum3/1
  Divide/1 -> Sum3/2
  Sum3/1 -> Mux/1, Mux/2, Mux/3, Mux/4
  Demux/10 -> Terminato5/1
  Demux/11 -> Terminato6/1
  Demux/12 -> Terminato7/1
  Demux/13 -> Terminato8/1
  Demux/14 -> Terminato9/1
  Demux/15 -> Terminato10/1
  Saturation/1 -> Divide/2
  Mux1/1 -> z/1
  Thrust Multiplier/1 -> Fcn/1
  Mux/1 -> Product1/1
  Fcn/1 -> Product1/2
  Product1/1 -> commands/1, z Command/1

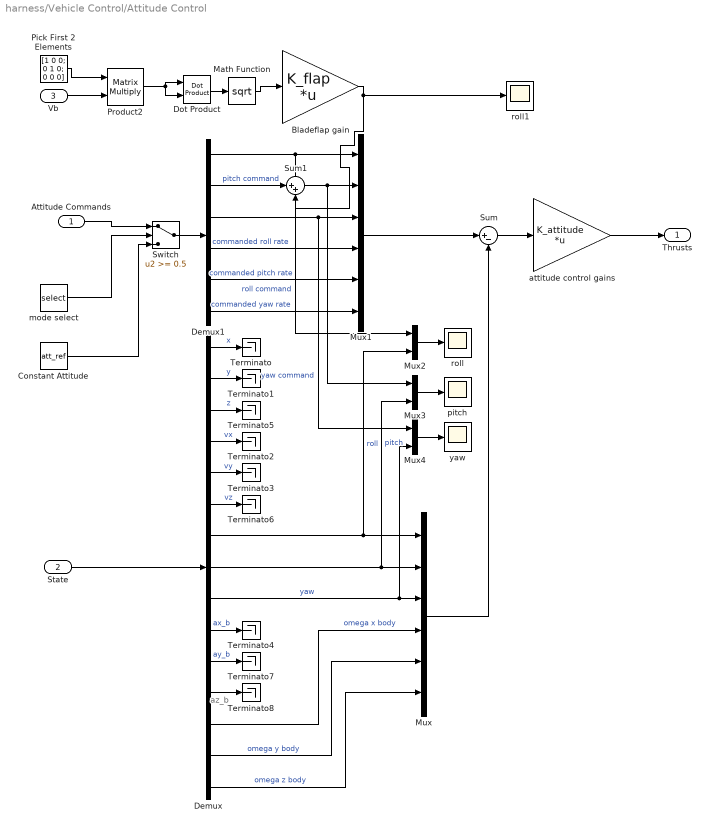
== system harness/Vehicle Control/Attitude Control ==
  note: az_b
  Attitude Commands : Inport  OutDataType=sfix(16)  OutScaling=2^0
  State : Inport  Port=2  OutDataType=sfix(16)  OutScaling=2^0
  Vb : Inport  Port=3  OutDataType=sfix(16)  OutScaling=2^0
  Bladeflap gain : Gain  Gain=K_flap  Multiplication=Matrix(K*u)  ParameterDataType=sfix(16)  ParameterScaling=2^0  OutDataType=sfix(16)  OutScaling=2^0
  Constant Attitude : Constant  Value=att_ref  OutDataType=sfix(16)  OutScaling=2^0
  Demux : Demux  Outputs=15
  Demux1 : Demux  Outputs=6
  Dot Product : simulink/Math Operations/Dot Product  InputSameDT=on  OutDataType=sfix(16)  OutScaling=2^-10  DoSatur=off
  Math Function : Math  Operator=sqrt  OutDataType=sfix(16)  OutScaling=2^0  SaturateOnIntegerOverflow=on
  Mux : Mux  Inputs=6
  Mux1 : Mux  Inputs=6
  Mux2 : Mux  Inputs=2
  Mux3 : Mux  Inputs=2
  Mux4 : Mux  Inputs=2
  Pick First 2 Elements : Constant  Value=[1 0 0; 0 1 0; 0 0 0]  OutDataType=sfix(16)  OutScaling=2^0
  Product2 : Product  Multiplication=Matrix(*)  OutDataType=sfix(16)  OutScaling=2^0  RndMeth=Zero
  Sum : Sum  Inputs=|+-  OutDataType=sfix(16)  OutScaling=2^0
  Sum1 : Sum  Inputs=|++  OutDataType=sfix(16)  OutScaling=2^0
  Switch : Switch  Threshold=0.5
  Terminato{,1..8} (9 alike) : Terminator
  attitude control gains : Gain  Gain=K_attitude  Multiplication=Matrix(K*u)  ParameterDataType=sfix(16)  ParameterScaling=2^0  OutDataType=sfix(16)  OutScaling=2^0
  mode select : Constant  Value=select  OutDataType=sfix(16)  OutScaling=2^0
  pitch : Scope
      settings: YMin=-0.01  YMax=0.11
  roll : Scope
      settings: YMin=-0.02  YMax=0.1
  roll1 : Scope
      settings: YMin=-0.02  YMax=0.1  SaveName=ScopeData21
  yaw : Scope
      settings: YMin=-0.25  YMax=0.3  SaveName=ScopeData2
  Thrusts : Outport  OutDataType=sfix(16)  OutScaling=2^0
  wires:
  Demux/1 -> Terminato/1  "x"
  Demux/2 -> Terminato1/1  "y"
  Demux/5 -> Terminato3/1  "vy"
  Demux/4 -> Terminato2/1  "vx"
  Demux/7 -> Mux/1, Mux2/2  "roll"
  Demux/8 -> Mux/2, Mux3/2  "pitch"
  Demux/9 -> Mux/3, Mux4/2  "yaw"
  State/1 -> Demux/1
  Demux/3 -> Terminato5/1  "z"
  Demux/6 -> Terminato6/1  "vz"
  Demux/10 -> Terminato4/1  "ax_b"
  Demux/11 -> Terminato7/1  "ay_b"
  Demux/12 -> Terminato8/1
  Demux/13 -> Mux/4  "omega x body"
  Demux/14 -> Mux/5  "omega y body"
  Demux/15 -> Mux/6  "omega z body"
  Demux1/1 -> Mux1/1, Mux2/1  "roll command"
  Demux1/2 -> Sum1/1  "pitch command"
  Demux1/3 -> Mux1/3, Mux4/1  "yaw command"
  Demux1/4 -> Mux1/4  "commanded roll rate"
  Demux1/5 -> Mux1/5  "commanded pitch rate"
  Demux1/6 -> Mux1/6  "commanded yaw rate"
  Mux1/1 -> Sum/1
  Mux/1 -> Sum/2
  Sum/1 -> attitude control gains/1
  attitude control gains/1 -> Thrusts/1
  mode select/1 -> Switch/2
  Constant Attitude/1 -> Switch/3
  Switch/1 -> Demux1/1
  Mux4/1 -> yaw/1
  Mux3/1 -> pitch/1
  Mux2/1 -> roll/1
  Attitude Commands/1 -> Switch/1
  Pick First 2 Elements/1 -> Product2/1
  Vb/1 -> Product2/2
  Dot Product/1 -> Math Function/1
  Product2/1 -> Dot Product/1, Dot Product/2
  Math Function/1 -> Bladeflap gain/1
  Bladeflap gain/1 -> Sum1/2, roll1/1
  Sum1/1 -> Mux1/2, Mux3/1

== system harness/Vehicle Control/Position Control ==
  state : Inport  OutDataType=sfix(16)  OutScaling=2^0
  Constant Attitude : Constant  Value=att_ref  OutDataType=sfix(16)  OutScaling=2^0
  Demux : Demux  Outputs=15
  Mux : Mux  Inputs=13
  Terminato : Terminator
  Terminato1 : Terminator
  Terminato2 : Terminator
  Attitude : Outport  OutDataType=sfix(16)  OutScaling=2^0
  wires:
  Constant Attitude/1 -> Attitude/1
  state/1 -> Demux/1
  Demux/1 -> Terminato2/1
  Demux/2 -> Terminato1/1
  Demux/3 -> Mux/1
  Demux/4 -> Mux/2
  Demux/5 -> Mux/3
  Demux/6 -> Mux/4
  Demux/7 -> Mux/5
  Demux/8 -> Mux/6
  Demux/9 -> Mux/7
  Demux/10 -> Mux/8
  Demux/11 -> Mux/9
  Demux/12 -> Mux/10
  Demux/13 -> Mux/11
  Demux/14 -> Mux/12
  Demux/15 -> Mux/13
  Mux/1 -> Terminato/1

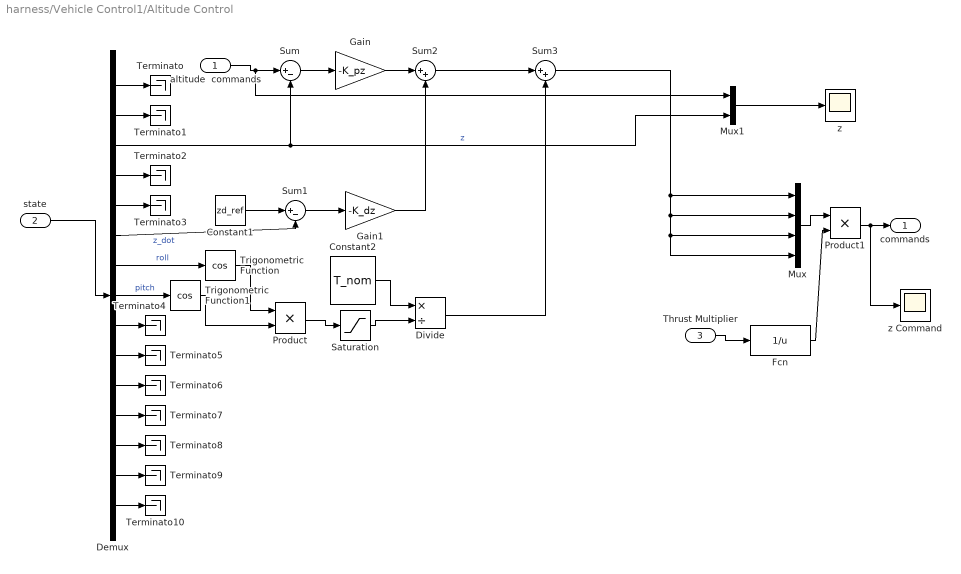
== system harness/Vehicle Control1/Altitude Control ==
  altitude  commands : Inport  OutDataType=sfix(16)  OutScaling=2^0
  state : Inport  Port=2  OutDataType=sfix(16)  OutScaling=2^0
  Thrust Multiplier : Inport  Port=3  OutDataType=sfix(16)  OutScaling=2^0
  Constant1 : Constant  Value=zd_ref  OutDataType=sfix(16)  OutScaling=2^0
  Constant2 : Constant  Value=T_nom  OutDataType=sfix(16)  OutScaling=2^0
  Demux : Demux  Outputs=15
  Divide : Product  Inputs=*/  OutDataType=sfix(16)  OutScaling=2^-10
  Fcn : Fcn  Expr=1/u
  Gain : Gain  Gain=-K_pz  ParameterDataType=sfix(16)  ParameterScaling=2^0  OutDataType=sfix(16)  OutScaling=2^0
  Gain1 : Gain  Gain=-K_dz  ParameterDataType=sfix(16)  ParameterScaling=2^0  OutDataType=sfix(16)  OutScaling=2^0
  Mux : Mux
  Mux1 : Mux  Inputs=2
  Product : Product  OutDataType=sfix(16)  OutScaling=2^0  RndMeth=Zero
  Product1 : Product  OutDataType=sfix(16)  OutScaling=2^0  RndMeth=Zero
  Saturation : Saturate  UpperLimit=1  LowerLimit=0.01
  Sum : Sum  Inputs=|+-  OutDataType=sfix(16)  OutScaling=2^0
  Sum1 : Sum  Inputs=|+-  OutDataType=sfix(16)  OutScaling=2^0
  Sum2 : Sum  Inputs=|++  OutDataType=sfix(16)  OutScaling=2^0
  Sum3 : Sum  Inputs=|++  OutDataType=sfix(16)  OutScaling=2^0
  Terminato{,1..10} (11 alike) : Terminator
  Trigonometric Function : Trigonometry  Operator=cos
  Trigonometric Function1 : Trigonometry  Operator=cos
  z : Scope
      settings: SaveName=ScopeData3
  z Command : Scope
      settings: SaveName=ScopeData5
  commands : Outport  OutDataType=sfix(16)  OutScaling=2^0
  wires:
  state/1 -> Demux/1
  Demux/1 -> Terminato/1
  Demux/2 -> Terminato1/1
  Demux/5 -> Terminato3/1
  Demux/4 -> Terminato2/1
  Demux/3 -> Sum/2, Mux1/2  "z"
  altitude  commands/1 -> Sum/1, Mux1/1
  Constant1/1 -> Sum1/1
  Demux/6 -> Sum1/2  "z_dot"
  Sum/1 -> Gain/1
  Sum1/1 -> Gain1/1
  Gain/1 -> Sum2/1
  Gain1/1 -> Sum2/2
  Demux/7 -> Trigonometric Function/1  "roll"
  Demux/8 -> Trigonometric Function1/1  "pitch"
  Demux/9 -> Terminato4/1
  Trigonometric Function/1 -> Product/1
  Trigonometric Function1/1 -> Product/2
  Product/1 -> Saturation/1
  Constant2/1 -> Divide/1
  Sum2/1 -> Sum3/1
  Divide/1 -> Sum3/2
  Sum3/1 -> Mux/1, Mux/2, Mux/3, Mux/4
  Demux/10 -> Terminato5/1
  Demux/11 -> Terminato6/1
  Demux/12 -> Terminato7/1
  Demux/13 -> Terminato8/1
  Demux/14 -> Terminato9/1
  Demux/15 -> Terminato10/1
  Saturation/1 -> Divide/2
  Mux1/1 -> z/1
  Thrust Multiplier/1 -> Fcn/1
  Mux/1 -> Product1/1
  Fcn/1 -> Product1/2
  Product1/1 -> commands/1, z Command/1

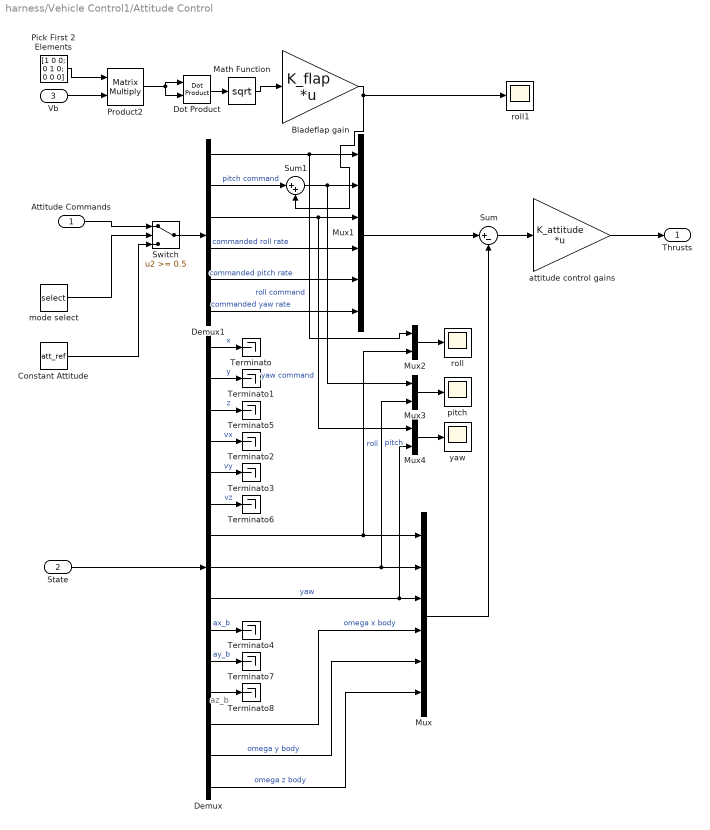
== system harness/Vehicle Control1/Attitude Control ==
  note: az_b
  Attitude Commands : Inport  OutDataType=sfix(16)  OutScaling=2^0
  State : Inport  Port=2  OutDataType=sfix(16)  OutScaling=2^0
  Vb : Inport  Port=3  OutDataType=sfix(16)  OutScaling=2^0
  Bladeflap gain : Gain  Gain=K_flap  Multiplication=Matrix(K*u)  ParameterDataType=sfix(16)  ParameterScaling=2^0  OutDataType=sfix(16)  OutScaling=2^0
  Constant Attitude : Constant  Value=att_ref  OutDataType=sfix(16)  OutScaling=2^0
  Demux : Demux  Outputs=15
  Demux1 : Demux  Outputs=6
  Dot Product : simulink/Math Operations/Dot Product  InputSameDT=on  OutDataType=sfix(16)  OutScaling=2^-10  DoSatur=off
  Math Function : Math  Operator=sqrt  OutDataType=sfix(16)  OutScaling=2^0  SaturateOnIntegerOverflow=on
  Mux : Mux  Inputs=6
  Mux1 : Mux  Inputs=6
  Mux2 : Mux  Inputs=2
  Mux3 : Mux  Inputs=2
  Mux4 : Mux  Inputs=2
  Pick First 2 Elements : Constant  Value=[1 0 0; 0 1 0; 0 0 0]  OutDataType=sfix(16)  OutScaling=2^0
  Product2 : Product  Multiplication=Matrix(*)  OutDataType=sfix(16)  OutScaling=2^0  RndMeth=Zero
  Sum : Sum  Inputs=|+-  OutDataType=sfix(16)  OutScaling=2^0
  Sum1 : Sum  Inputs=|++  OutDataType=sfix(16)  OutScaling=2^0
  Switch : Switch  Threshold=0.5
  Terminato{,1..8} (9 alike) : Terminator
  attitude control gains : Gain  Gain=K_attitude  Multiplication=Matrix(K*u)  ParameterDataType=sfix(16)  ParameterScaling=2^0  OutDataType=sfix(16)  OutScaling=2^0
  mode select : Constant  Value=select  OutDataType=sfix(16)  OutScaling=2^0
  pitch : Scope
      settings: YMin=-0.01  YMax=0.11
  roll : Scope
      settings: YMin=-0.02  YMax=0.1
  roll1 : Scope
      settings: YMin=-0.02  YMax=0.1  SaveName=ScopeData21
  yaw : Scope
      settings: YMin=-0.25  YMax=0.3  SaveName=ScopeData2
  Thrusts : Outport  OutDataType=sfix(16)  OutScaling=2^0
  wires:
  Demux/1 -> Terminato/1  "x"
  Demux/2 -> Terminato1/1  "y"
  Demux/5 -> Terminato3/1  "vy"
  Demux/4 -> Terminato2/1  "vx"
  Demux/7 -> Mux/1, Mux2/2  "roll"
  Demux/8 -> Mux/2, Mux3/2  "pitch"
  Demux/9 -> Mux/3, Mux4/2  "yaw"
  State/1 -> Demux/1
  Demux/3 -> Terminato5/1  "z"
  Demux/6 -> Terminato6/1  "vz"
  Demux/10 -> Terminato4/1  "ax_b"
  Demux/11 -> Terminato7/1  "ay_b"
  Demux/12 -> Terminato8/1
  Demux/13 -> Mux/4  "omega x body"
  Demux/14 -> Mux/5  "omega y body"
  Demux/15 -> Mux/6  "omega z body"
  Demux1/1 -> Mux1/1, Mux2/1  "roll command"
  Demux1/2 -> Sum1/1  "pitch command"
  Demux1/3 -> Mux1/3, Mux4/1  "yaw command"
  Demux1/4 -> Mux1/4  "commanded roll rate"
  Demux1/5 -> Mux1/5  "commanded pitch rate"
  Demux1/6 -> Mux1/6  "commanded yaw rate"
  Mux1/1 -> Sum/1
  Mux/1 -> Sum/2
  Sum/1 -> attitude control gains/1
  attitude control gains/1 -> Thrusts/1
  mode select/1 -> Switch/2
  Constant Attitude/1 -> Switch/3
  Switch/1 -> Demux1/1
  Mux4/1 -> yaw/1
  Mux3/1 -> pitch/1
  Mux2/1 -> roll/1
  Attitude Commands/1 -> Switch/1
  Pick First 2 Elements/1 -> Product2/1
  Vb/1 -> Product2/2
  Dot Product/1 -> Math Function/1
  Product2/1 -> Dot Product/1, Dot Product/2
  Math Function/1 -> Bladeflap gain/1
  Bladeflap gain/1 -> Sum1/2, roll1/1
  Sum1/1 -> Mux1/2, Mux3/1

== system harness/Vehicle Control1/Position Control ==
  state : Inport  OutDataType=sfix(16)  OutScaling=2^0
  Constant Attitude : Constant  Value=att_ref  OutDataType=sfix(16)  OutScaling=2^0
  Demux : Demux  Outputs=15
  Mux : Mux  Inputs=13
  Terminato : Terminator
  Terminato1 : Terminator
  Terminato2 : Terminator
  Attitude : Outport  OutDataType=sfix(16)  OutScaling=2^0
  wires:
  Constant Attitude/1 -> Attitude/1
  state/1 -> Demux/1
  Demux/1 -> Terminato2/1
  Demux/2 -> Terminato1/1
  Demux/3 -> Mux/1
  Demux/4 -> Mux/2
  Demux/5 -> Mux/3
  Demux/6 -> Mux/4
  Demux/7 -> Mux/5
  Demux/8 -> Mux/6
  Demux/9 -> Mux/7
  Demux/10 -> Mux/8
  Demux/11 -> Mux/9
  Demux/12 -> Mux/10
  Demux/13 -> Mux/11
  Demux/14 -> Mux/12
  Demux/15 -> Mux/13
  Mux/1 -> Terminato/1

== system harness/Wind Model/Single Wind Gust Model ==
  Enable : EnablePort
  Clock : Clock
      settings: Decimation=10
  Constant : Constant  OutDataType=sfix(16)  OutScaling=2^0
  Constant1 : Constant  Value=wind_start  OutDataType=sfix(16)  OutScaling=2^0
  Constant2 : Constant  Value=0.5*wind_max  OutDataType=sfix(16)  OutScaling=2^0
  Frequency : Constant  Value=2*pi/wind_duration  OutDataType=sfix(16)  OutScaling=2^0
  Mux : Mux  Inputs=3
  Product : Product  OutDataType=sfix(16)  OutScaling=2^0  RndMeth=Zero
  Product1 : Product  OutDataType=sfix(16)  OutScaling=2^0  RndMeth=Zero
  Product2 : Product  OutDataType=sfix(16)  OutScaling=2^0  RndMeth=Zero
  Random Number : RandomNumber  Variance=wind_var  Seed=w_seed  SampleTime=t_s
  Random Number1 : RandomNumber  Variance=wind_var  Seed=w_seed+1  SampleTime=t_s
  Random Number2 : RandomNumber  Variance=wind_var  Seed=w_seed+2  SampleTime=t_s
  Saturation : Saturate  UpperLimit=wind_clip  LowerLimit=0
  Sum : Sum  Inputs=|+-  OutDataType=sfix(16)  OutScaling=2^0
  Sum1 : Sum  Inputs=|+-  OutDataType=sfix(16)  OutScaling=2^0
  Sum2 : Sum  Inputs=|++  OutDataType=sfix(16)  OutScaling=2^0
  Trigonometric Function : Trigonometry  Operator=cos
  Wind Vector : Constant  Value=wind_vector  OutDataType=sfix(16)  OutScaling=2^0
  Wind Velocity : Outport  OutDataType=sfix(16)  OutScaling=2^0
  wires:
  Constant/1 -> Sum/1
  Wind Vector/1 -> Product/1
  Trigonometric Function/1 -> Sum/2
  Frequency/1 -> Product1/2
  Product1/1 -> Trigonometric Function/1
  Clock/1 -> Sum1/1
  Constant1/1 -> Sum1/2
  Sum1/1 -> Product1/1
  Sum/1 -> Product2/1
  Constant2/1 -> Product2/2
  Product2/1 -> Saturation/1
  Saturation/1 -> Product/2
  Random Number/1 -> Mux/1
  Random Number1/1 -> Mux/2
  Random Number2/1 -> Mux/3
  Product/1 -> Sum2/1
  Sum2/1 -> Wind Velocity/1
  Mux/1 -> Sum2/2

== system harness/Wind Model1/Single Wind Gust Model ==
  Enable : EnablePort
  Clock : Clock
      settings: Decimation=10
  Constant : Constant  OutDataType=sfix(16)  OutScaling=2^0
  Constant1 : Constant  Value=wind_start  OutDataType=sfix(16)  OutScaling=2^0
  Constant2 : Constant  Value=0.5*wind_max  OutDataType=sfix(16)  OutScaling=2^0
  Frequency : Constant  Value=2*pi/wind_duration  OutDataType=sfix(16)  OutScaling=2^0
  Mux : Mux  Inputs=3
  Product : Product  OutDataType=sfix(16)  OutScaling=2^0  RndMeth=Zero
  Product1 : Product  OutDataType=sfix(16)  OutScaling=2^0  RndMeth=Zero
  Product2 : Product  OutDataType=sfix(16)  OutScaling=2^0  RndMeth=Zero
  Random Number : RandomNumber  Variance=wind_var  Seed=w_seed  SampleTime=t_s
  Random Number1 : RandomNumber  Variance=wind_var  Seed=w_seed+1  SampleTime=t_s
  Random Number2 : RandomNumber  Variance=wind_var  Seed=w_seed+2  SampleTime=t_s
  Saturation : Saturate  UpperLimit=wind_clip  LowerLimit=0
  Sum : Sum  Inputs=|+-  OutDataType=sfix(16)  OutScaling=2^0
  Sum1 : Sum  Inputs=|+-  OutDataType=sfix(16)  OutScaling=2^0
  Sum2 : Sum  Inputs=|++  OutDataType=sfix(16)  OutScaling=2^0
  Trigonometric Function : Trigonometry  Operator=cos
  Wind Vector : Constant  Value=wind_vector  OutDataType=sfix(16)  OutScaling=2^0
  Wind Velocity : Outport  OutDataType=sfix(16)  OutScaling=2^0
  wires:
  Constant/1 -> Sum/1
  Wind Vector/1 -> Product/1
  Trigonometric Function/1 -> Sum/2
  Frequency/1 -> Product1/2
  Product1/1 -> Trigonometric Function/1
  Clock/1 -> Sum1/1
  Constant1/1 -> Sum1/2
  Sum1/1 -> Product1/1
  Sum/1 -> Product2/1
  Constant2/1 -> Product2/2
  Product2/1 -> Saturation/1
  Saturation/1 -> Product/2
  Random Number/1 -> Mux/1
  Random Number1/1 -> Mux/2
  Random Number2/1 -> Mux/3
  Product/1 -> Sum2/1
  Sum2/1 -> Wind Velocity/1
  Mux/1 -> Sum2/2

== system harness/Subsystem/6DOF (Euler Angles)_CMU/Body-based-to-ref-frame-based ==
  note: dF/dt = P + Q sinF tanQ + R cosF tanQ
      | dQ/dt = Q cosF - R sinF
      | dY/dt = Q sinF secQ + R cosF secQ
  omega : Inport  OutDataType=sfix(16)  OutScaling=2^0
  theta : Inport  Port=2  OutDataType=sfix(16)  OutScaling=2^0
  Fcn : Fcn  Expr=u[1]+u[2]*sin(u[4])*tan(u[5])+u[3]*cos(u[4])*tan(u[5])
  Fcn1 : Fcn  Expr=u[2]*cos(u[4])-u[3]*sin(u[4])
  Fcn2 : Fcn  Expr=u[2]*sin(u[4])*(1/cos(u[5]))+u[3]*cos(u[4])*(1/cos(u[5]))
  Mux : Mux  Inputs=2
  Mux1 : Mux  Inputs=3
  Out1 : Outport  OutDataType=sfix(16)  OutScaling=2^0
  wires:
  Mux1/1 -> Out1/1
  Fcn2/1 -> Mux1/3
  Fcn1/1 -> Mux1/2
  Fcn/1 -> Mux1/1
  Mux/1 -> Fcn2/1, Fcn1/1, Fcn/1
  theta/1 -> Mux/2
  omega/1 -> Mux/1
